simulink model "SurgeArrester"  (R2020a)
settings: Solver=VariableStepAuto  StartTime=0.0  StopTime=0.25  RelTol=1e-3
libraries: powerlib x18, powerlib_meascontrol x2
settings Model: Creator=Alisamar  LastModifiedBy=Alisamar
settings SolverCC: ZeroCrossAlgorithm=Adaptive
settings DebuggingCC: IgnoredZcDiagnostic=none

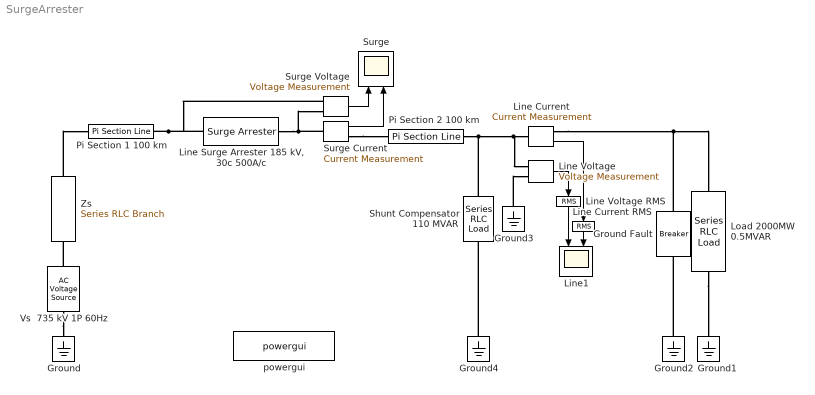
== system SurgeArrester ==
  Ground{,1..4} (5 alike) : powerlib/Elements/Ground  LConnTagsString=a
  Ground Fault : powerlib/Elements/Breaker  InitialState=0  SwitchingTimes="[5/60  10/60]"  External=off  BreakerResistance=0.01  SnubberResistance=100e6  SnubberCapacitance=0  Measurements=None  MoreParameters=on  NoBreakLoop=off
  Line Current : powerlib/Measurements/Current Measurement  PhasorSimulation=off  OutputType=Complex  PSBequivalent=0
  Line Current RMS : powerlib_meascontrol/Measurements/RMS  TrueRMS=on  Freq=60  RMSInit=120  Ts=0
  "Line Surge Arrester 185 kV, 30c 500A/c" : powerlib/Elements/Surge Arrester  ProtectionVoltage=185e3  Columns=30  ReferenceCurrent=500  Segment1=[.955 50]  Segment2=[1.0 25]  Segment3=[.9915 16.5]  Measurements=None  BreakLoop=off  UseDiscreteRobustSolver=on
      settings: SourceProductBaseCode=PS
  Line Voltage : powerlib/Measurements/Voltage Measurement  PhasorSimulation=off  OutputType=Complex  PSBequivalent=0
  Line Voltage RMS : powerlib_meascontrol/Measurements/RMS  TrueRMS=on  Freq=60  RMSInit=120  Ts=0
  Line1 : Scope  NumInputPorts=2
  Load 2000MW 0.5MVAR : powerlib/Elements/Series RLC Load  LConnTagsString=a  RConnTagsString=__new0  NominalVoltage=100e3  NominalFrequency=60  ActivePower=2000e6  InductivePower=0.5e6  CapacitivePower=0  Setx0=off  InitialVoltage=0  SetiL0=off  InitialCurrent=0  Measurements=None  LoadType=constant Z
  Pi Section 1 100 km : powerlib/Elements/Pi Section Line  LConnTagsString=__new0  RConnTagsString=__new0  Frequency=60  Resistance=0.01273  Inductance=0.9337e-3  Capacitance=12.74e-9  Length=100  PiSections=1  Measurements=None
      settings: AttributesFormatString=\n  SourceProductBaseCode=PS
  Pi Section 2 100 km : powerlib/Elements/Pi Section Line  LConnTagsString=__new0  RConnTagsString=__new0  Frequency=60  Resistance=0.01273  Inductance=0.9337e-3  Capacitance=12.74e-9  Length=100  PiSections=1  Measurements=None
      settings: AttributesFormatString=\n  SourceProductBaseCode=PS
  Shunt Compensator 110 MVAR : powerlib/Elements/Series RLC Load  LConnTagsString=a  RConnTagsString=__new0  NominalVoltage=1000  NominalFrequency=60  ActivePower=0  InductivePower=110e6  CapacitivePower=0  Setx0=off  InitialVoltage=0  SetiL0=off  InitialCurrent=0  Measurements=None  LoadType=constant Z
  Surge : Scope  NumInputPorts=2
  Surge Current : powerlib/Measurements/Current Measurement  PhasorSimulation=off  OutputType=Complex  PSBequivalent=0
  Surge Voltage : powerlib/Measurements/Voltage Measurement  PhasorSimulation=off  OutputType=Complex  PSBequivalent=0
  Vs  735 kV 1P 60Hz : powerlib/Electrical Sources/AC Voltage Source  Amplitude=735e3  Phase=0  Frequency=60  SampleTime=0  Measurements=None  BusType=swing  Pref=10e3  Qref=0  Qmin=-inf  Qmax=+inf
  Zs : powerlib/Elements/Series RLC Branch  LConnTagsString=__new0  RConnTagsString=__new0  BranchType=RL  Resistance=1  Inductance=1e-3  SetiL0=off  InitialCurrent=0  Capacitance=1e-6  Setx0=off  InitialVoltage=0  Measurements=None
  powergui : powerlib/powergui  Priority=1  SimulationMode=Continuous  SampleTime=50e-6  frequency=60  Iterations=50  frequencyindice=60  Pbase=100e6  ErrMax=1e-4  UnitsV=kV  UnitsW=MW  buscounter=0  FunctionMessages=off  echomessages=off  EnableUseOfTLC=off  CurrentSourceSwitches=off  DisableSnubberDevices=off  DisableRonSwitches=off  DisableVfSwitches=off  DisplayEquations=off  AutomaticDiscreteSolvers=off  SolverType=Tustin/Backward Euler (TBE)  Interpol=off  ExternalGateDelay=off  methode=off  Ts=100  x0status=blocks  SPID=on  SwTol=0  HookPort=off  NonlinearTolerance=1e-4  nMaxIteration=100  ContinueOnMaxIteration=off  RestoreLinks=warning  ResistiveCurrentMeasurement=off  Frange=[0:2:500]  Ylog=off  Xlog=on  ShowGrid=off  save=off  variable=ZData  structure=0  ZoomFFT=off  StartTime=0.0  cycles=1  DisplayStyle=1  fundamental=60  FreqAxis=off  MaxFrequency=1000  frequencyindicesteady=1  RmsSteady=1  display=off
  wires:
  Surge Voltage/1 -> Surge/1
  Surge Current/1 -> Surge/2
  Line Current/1 -> Line Current RMS/1
  Line Voltage/1 -> Line Voltage RMS/1
  Line Current RMS/1 -> Line1/2
  Line Voltage RMS/1 -> Line1/1
  connections:
  Vs  735 kV 1P 60Hz/RConn1 -- Zs/LConn1
  Vs  735 kV 1P 60Hz/LConn1 -- Ground/LConn1
  Zs/RConn1 -- Pi Section 1 100 km/LConn1
  Ground Fault/LConn1 -- Line Current/RConn1 -- Load 2000MW 0.5MVAR/LConn1
  Surge Current/RConn1 -- Pi Section 2 100 km/LConn1
  Pi Section 1 100 km/RConn1 -- Surge Voltage/LConn1 -- "Line Surge Arrester 185 kV, 30c 500A/c"/LConn1
  Load 2000MW 0.5MVAR/RConn1 -- Ground1/LConn1
  Surge Current/LConn1 -- Surge Voltage/LConn2 -- "Line Surge Arrester 185 kV, 30c 500A/c"/RConn1
  Pi Section 2 100 km/RConn1 -- Line Voltage/LConn1 -- Line Current/LConn1 -- Shunt Compensator 110 MVAR/RConn1
  Ground2/LConn1 -- Ground Fault/RConn1
  Ground4/LConn1 -- Shunt Compensator 110 MVAR/LConn1
  Ground3/LConn1 -- Line Voltage/LConn2
